simulink model "control"  (R2017b)
settings: Solver=VariableStepAuto  StartTime=0.0  StopTime=10.0  RelTol=1e-3
libraries: instrumentlib x2
settings Model: Creator=Zhenger  LastModifiedBy=Zhenger

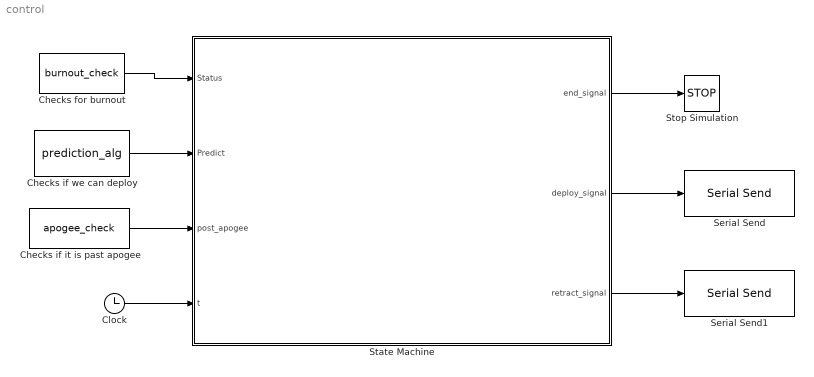
== system control ==
  Checks for burnout : DataStoreRead  DataStoreName=burnout_check
  Checks if it is past apogee : DataStoreRead  DataStoreName=apogee_check
  Checks if we can deploy : DataStoreRead  DataStoreName=prediction_alg
  Clock : Clock
  Serial Send : instrumentlib/Serial Send  ComPortMenu=<Please select a port...>  ComPort=<Please select a port...>  Terminator=<none>  EnableBlockingMode=on
  Serial Send1 : instrumentlib/Serial Send  ComPortMenu=<Please select a port...>  ComPort=<Please select a port...>  Terminator=<none>  EnableBlockingMode=on
  State Machine : Stateflow chart  TreatAsAtomicUnit=on
  Stop Simulation : Stop
  wires:
  Clock/1 -> State Machine/4(t)
  Checks if we can deploy/1 -> State Machine/2(Predict)
  Checks for burnout/1 -> State Machine/1(Status)
  Checks if it is past apogee/1 -> State Machine/3(post_apogee)
  State Machine/1(end_signal) -> Stop Simulation/1
  State Machine/2(deploy_signal) -> Serial Send/1
  State Machine/3(retract_signal) -> Serial Send1/1

== stateflow chart control/State Machine ==
  state STANDBY
    entry:
    post_burnout = Status();
  state PREDICT_APOGEE
    entry:
    t=0;
    during:
    deploy=Predict();
  state DEPLOY_BRAKES
    entry:
    deploy_signal = Simulink.Signal
  state POST_APOGEE
    entry:
    end_signal = Simulink.Signal
  state RETRACT_BRAKES
    entry:
    retract_signal = Simulink.Signal
  (default) -> STANDBY
  STANDBY -> STANDBY [order 2]
  STANDBY -> PREDICT_APOGEE [order 1] : [post_burnout == 1]
  PREDICT_APOGEE -> PREDICT_APOGEE [order 2] : [post_apogee == 0]
  PREDICT_APOGEE -> POST_APOGEE [order 3] : [post_apogee == 1]
  PREDICT_APOGEE -> DEPLOY_BRAKES [order 1] : [deploy == 1]
  DEPLOY_BRAKES -> RETRACT_BRAKES : after(3, sec)
  data: Status input; Predict input; post_apogee input; t input; end_signal output; deploy_signal output; retract_signal output; deploy local; post_burnout local
